simulink model "TestModel_V2_2024a"  (R2024a)
settings: Solver=FixedStepAuto  StartTime=0.0  StopTime=40  FixedStep=1e-6  RelTol=1e-3
values from neighbouring files (symbols this model uses):
  pmsm = mcb.getPMSMParameters('Teknic2310P')    [mcb_pmsm_foc_sensorless_f28379d_datascript.m]
  Ts = T_pwm    (= 5e-05)    [mcb_pmsm_foc_sensorless_f28379d_datascript.m]
  Ts_motor = T_pwm/2    (= 2.5e-05)    [mcb_pmsm_foc_sensorless_f28379d_datascript.m]
undefined symbols (not defined in the file or in its folder): DiscIntNeverNeededParam, IM, par_Ctrl_SpdRt
libraries: mcbcontrolslib x7, spsOnDelayLib x6, autolibim x3, spsCurrentMeasurementLib x2, spsDCVoltageSourceLib x2, spsVoltageMeasurementLib x2, spsTwoLevelConverterLib x2, spsThreePhaseVIMeasurementLib x2, spsTriangleGeneratorLib x2, spsUniversalBridgeLib x1, autolibpmsminterior x1, eePwmGeneratorTwoLevel x1
settings Model: SimulationMode=accelerator  PacingRate=1000  Creator=ckb527612  LastModifiedBy=ckb527612
settings ConfigComp: CovBoundaryAbsTol=1.0e-5
settings SimscapeCC: EditingMode=Restricted

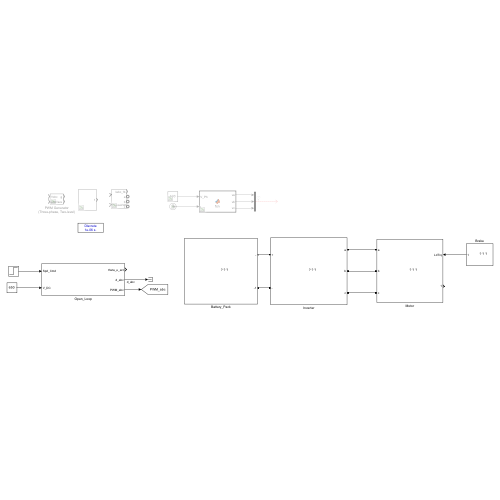
[thumbnail: Simulink's stored preview of the top-level diagram]
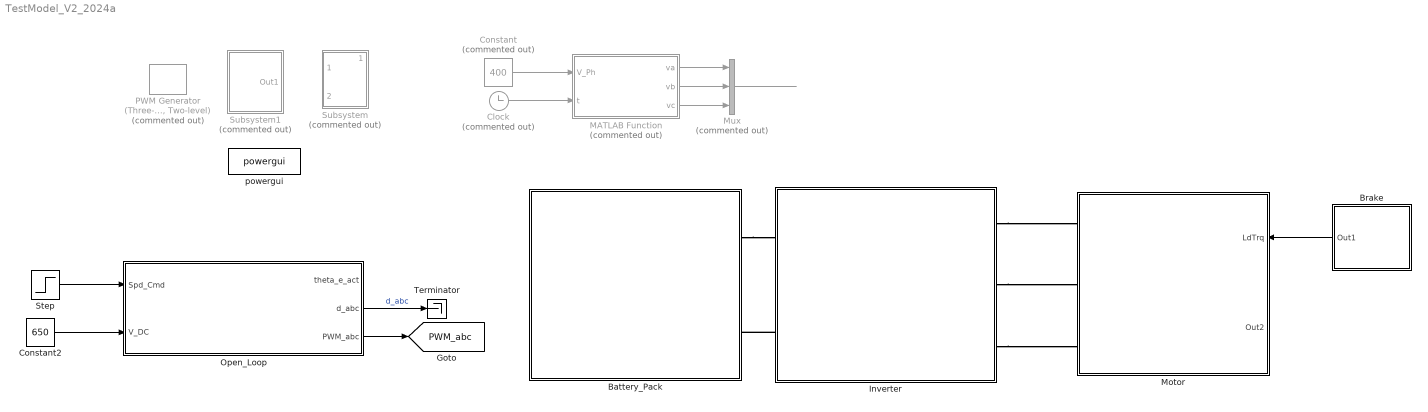
== system TestModel_V2_2024a ==
  Battery_Pack : Subsystem
      mask Display: image('battery_pack.jpg');
  Brake : Subsystem
      mask Display: image('brake-system-types-and-hydraulic-brake-parts-and-functions-6.png');
  Clock : Clock  Commented=on
  Constant : Constant  Commented=on  Value=400
  Constant2 : Constant  Value=650
  Inverter : Subsystem
      mask Display: image('inverter.jpg');
  MATLAB Function : MATLAB Function  Commented=on  TreatAsAtomicUnit=on
  Motor : Subsystem
      settings: PortSchema="{\"entries\":[{\"content\":{\"sides\":[{\"content\":{\"connectorIds\":[\"LConn1\",\"LConn2\",\"LConn3\"]},\"type\":\"ConnectorPlacement.EquallySpacedRectSide\",\"uuid\":\"ba224176-031b-46fb-9c66-bda2665a14bd\"},{\"content\":{\"connectorIds\":[\"In1\",\"Out1\"],\"side\":\"RIGHT\"},\"type\":\"ConnectorPlacement.EquallySpacedRectSide\",\"uuid\":\"afd0beac-69db-400a-8bb3-39f53f6dd0dc\"},{\"content\":{\"side\":\"TOP\"},\"type\":\"ConnectorPlacement.EquallySpacedRectSide\",\"uuid\":\"9d949d83-5907-4238-9cb9-0d10379fcdec\"}]},\"type\":\"ConnectorPlacement.EquallySpacedConnector\",\"uuid\":\"43d01ac6-0c0f-4af8-b336-a00f131902fe\"}],\"packageUris\":[\"http://schema.mathworks.com/mf0/Connector/R2020b\"],\"version\":\"1.0\"}"
      mask Display: image('Motor3.jpg');
  Mux : Mux  Commented=on  Inputs=3
  Open_Loop : Subsystem
  "PWM Generator (Three-phase, Two-level)" : eePwmGeneratorTwoLevel/PWM Generator (Three-phase, Two-level)  Commented=on  PWMMode=Continuous PWM (CPWM)  CPWMMode=SVM: space vector modulation  DPWMMode=60 DPWM: 60 degree discontinuous PWM  fsw=10e3  Ts=1e-6
      settings: LibrarySourceBlock=|
      | ee_sl_lib/Pulse Width
      | Modulation/PWM Generator
      | (Three-phase, Two-level)
  Step : Step  After=500
  Subsystem : Subsystem  Commented=on
  Subsystem1 : Subsystem  Commented=on
  Terminator : Terminator
  powergui : spspowerguiLib/powergui  Priority=1  SimulationMode=Discrete  SampleTime=1e-6  frequency=60  Iterations=50  frequencyindice=0  Pbase=100e6  ErrMax=1e-4  UnitsV=kV  UnitsW=MW  buscounter=0  FunctionMessages=off  echomessages=off  EnableUseOfTLC=off  CurrentSourceSwitches=off  DisableSnubberDevices=off  DisableRonSwitches=off  DisableVfSwitches=off  DisplayEquations=off  AutomaticDiscreteSolvers=off  SolverType=Tustin/Backward Euler (TBE)  Interpol=off  ExternalGateDelay=off  methode=off  Ts=100  x0status=blocks  SPID=on  SwTol=0  HookPort=off  NonlinearTolerance=1e-4  nMaxIteration=100  ContinueOnMaxIteration=off  RestoreLinks=warning  ResistiveCurrentMeasurement=off  Frange=[0:2:500]  Ylog=off  Xlog=on  ShowGrid=off  save=off  variable=ZData  structure=0  ZoomFFT=off  StartTime=0.0  cycles=1  DisplayStyle=1  fundamental=60  FreqAxis=off  MaxFrequency=1000  frequencyindicesteady=1  RmsSteady=1  display=off
  tag scope: PWM_abc=global
  wires:
  Constant/1 -> MATLAB Function/1(V_Ph)
  MATLAB Function/1(va) -> Mux/1
  MATLAB Function/2(vb) -> Mux/2
  MATLAB Function/3(vc) -> Mux/3
  Mux/1 -> ?
  Clock/1 -> MATLAB Function/2(t)
  Brake/1(Out1) -> Motor/1(LdTrq)
  Step/1 -> Open_Loop/1(Spd_Cmd)
  Constant2/1 -> Open_Loop/2(V_DC)
  Open_Loop/3(PWM_abc) -> [PWM_abc]
  Open_Loop/2(d_abc) -> Terminator/1  "d_abc"
  connections:
  Inverter/LConn2 -- Battery_Pack/RConn2
  Inverter/RConn2 -- Motor/LConn2
  Inverter/RConn1 -- Motor/LConn1
  Battery_Pack/RConn1 -- Inverter/LConn1
  Inverter/RConn3 -- Motor/LConn3

== system TestModel_V2_2024a/Battery_Pack ==
  Current Measurement : spsCurrentMeasurementLib/Current Measurement  PhasorSimulation=off  OutputType=Complex  PSBequivalent=0
  "V_in " : spsDCVoltageSourceLib/DC Voltage Source  Amplitude=650  Measurements=None
  Voltage Measurement : spsVoltageMeasurementLib/Voltage Measurement  PhasorSimulation=off  OutputType=Complex  PSBequivalent=0
  - : PMIOPort  Side=Right
  -1 : PMIOPort  Port=2  Side=Right
  tag scope: I_in=global, V_in=global
  wires:
  Current Measurement/1 -> [I_in]
  Voltage Measurement/1 -> [V_in]
  connections:
  Current Measurement/RConn1 -- -/RConn1
  Voltage Measurement/LConn1 -- Current Measurement/LConn1 -- "V_in "/RConn1
  "V_in "/LConn1 -- -1/RConn1 -- Voltage Measurement/LConn2

== system TestModel_V2_2024a/Brake ==
  Constant : Constant  Commented=on  Value=pmsm.LdTrq
  Data Type Conversion : DataTypeConversion  Commented=on  OutDataTypeStr=single  SaturateOnIntegerOverflow=off  RndMeth=Floor
  IIR Filter : mcbcontrolslib/IIR Filter  VariantControl=Low Pass Filter  VariantSelect=Low-pass  FilterConstantInputType=Specify via dialog  Filter_constant=0.001  InitialOutput=Specify via dialog  InitialOutputValue=0  ExternalReset=none  advancedSettings=off  Ts=50e-6  cutOff_freq=3.1863
  T_load : Step  Before=IM.Tshaft*0  After=IM.Tshaft*0.15  SampleTime=1e-6
  T_load1 : Step  Commented=on  Time=2.5  Before=pmsm.T_rated*0.1  After=pmsm.T_rated*0.5  SampleTime=Ts_motor
  Terminator : Terminator
  Out1 : Outport
  wires:
  Constant/1 -> Terminator/1
  T_load/1 -> IIR Filter/1
  IIR Filter/1 -> Out1/1

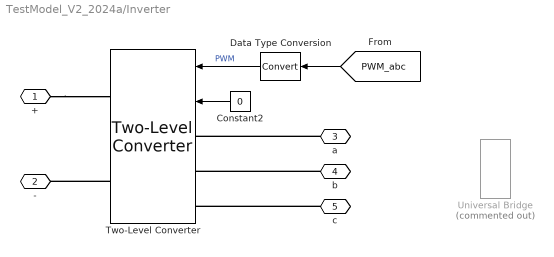
== system TestModel_V2_2024a/Inverter ==
  Constant2 : Constant  Value=0
  Data Type Conversion : DataTypeConversion  SaturateOnIntegerOverflow=off  RndMeth=Floor
  Two-Level Converter : spsTwoLevelConverterLib/Two-Level Converter  ModelType=Switching function  Ron=1e-3  Rs=1e6  Cs=inf  Vforward=[0,0]  Ron_Diode=1e-3  Rs_Diode=1e6  Cs_Diode=inf  Vf_Diode=0  Rs_CurrentSource=inf  Ron_ACsource=1e-3
  Universal Bridge : spsUniversalBridgeLib/Universal Bridge  Commented=on  Arms=3  SnubberResistance=1e5  SnubberCapacitance=inf  Device=IGBT / Diodes  Ron=1e-3  Lon=0  ForwardVoltages="[  0  0  ]"  ForwardVoltage=0  GTOparameters=[ 10e-6 , 20e-6 ]  IGBTparameters=[ 1e-6 , 2e-6 ]  Measurements=None  Measurements_2=None  converterType=Rectifier
  + : PMIOPort  Side=Left
  - : PMIOPort  Port=2  Side=Left
  a : PMIOPort  Port=3  Side=Right
  b : PMIOPort  Port=4  Side=Right
  c : PMIOPort  Port=5  Side=Right
  wires:
  Data Type Conversion/1 -> Two-Level Converter/1  "PWM"
  [PWM_abc] -> Data Type Conversion/1
  Constant2/1 -> Two-Level Converter/2
  connections:
  b/RConn1 -- Two-Level Converter/LConn2
  c/RConn1 -- Two-Level Converter/LConn3
  a/RConn1 -- Two-Level Converter/LConn1
  Two-Level Converter/RConn2 -- -/RConn1
  +/RConn1 -- Two-Level Converter/RConn1

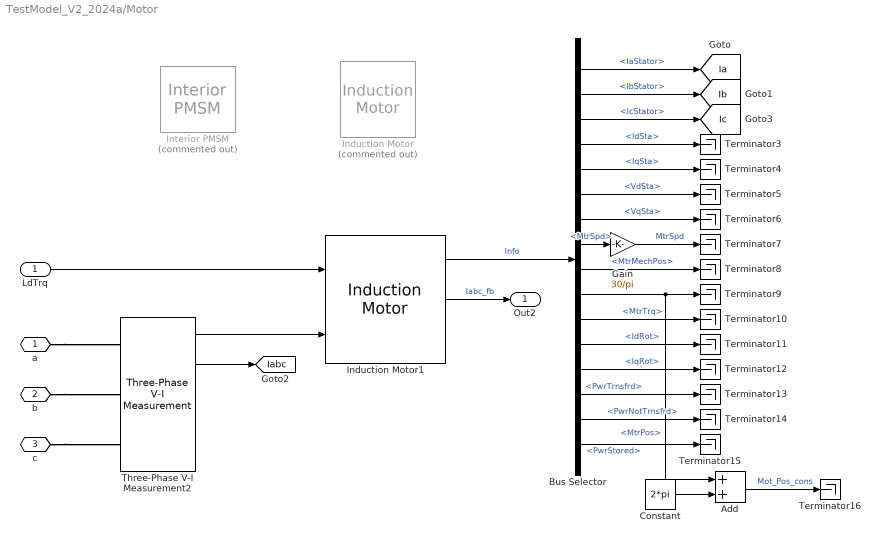
== system TestModel_V2_2024a/Motor ==
  LdTrq : Inport
  Add : Sum
  Bus Selector : BusSelector  OutputSignals=IaStator,IbStator,IcStator,IdSta,IqSta,VdSta,VqSta,MtrSpd,MtrMechPos,MtrPos,MtrTrq,IdRot,IqRot,PwrInfo.PwrTrnsfrd,PwrInfo.PwrNotTrnsfrd,PwrInfo.PwrStored
  Constant : Constant  Value=2*pi
  Gain : Gain  Gain=30/pi
  Induction Motor : autolibim/Induction Motor  Commented=on  sim_type=Discrete  Ts=0.001  port_config=Torque  P=2  Zs=[0.85 0.0139]  Zr="[0.55  0.0121]"  Lm=0.048  mechanical=[0.055 0.0078 0.5]  theta_init=0  omega_init=0  RefBlkName='autolibim/Induction Motor'  aMode=5
      settings: LibrarySourceBlock=mcblib/Electrical Systems/Motors/Induction Motor
  Induction Motor1 : autolibim/Induction Motor  sim_type=Discrete  Ts=1e-6  port_config=Torque  P=2  Zs=[3.14 0.0369]  Zr="[2.59  0.0369]"  Lm=0.527  mechanical=[0.01 0.00316 0.1]  theta_init=0  omega_init=0  RefBlkName='autolibim/Induction Motor'  aMode=5
      settings: LibrarySourceBlock=mcblib/Electrical Systems/Motors/Induction Motor
  Interior PMSM : autolibpmsminterior/Interior PMSM  Commented=on  port_config=Torque  sim_type=Continuous  Ts=0.001  FilePath=interiorpmsm_motordata.m  P=4  Rs=1.2  Ldq=[14.29e-3 23.15e-3]  KConstText=Permanent flux linkage constant (lambda_pm):  lambda_pm=0.5  Ke=159.9771  mechanical=[0.0045, 4.924e-4, 0]  idq0=[0 0]  theta_init=0  omega_init=0  KConst=0.1194  lambda_pm_calc=0.1194  Kt=1.323  RefBlkName='autolibpmsminterior/Interior PMSM'  aMode=1
      settings: LibrarySourceBlock=autolibemachines/Interior PMSM
  Terminator{3..16} (14 alike) : Terminator
  Three-Phase V-I Measurement2 : spsThreePhaseVIMeasurementLib/Three-Phase V-I Measurement  VoltageMeasurement=phase-to-phase  SetLabelV=off  LabelV=Vabc  Vpu=off  VpuLL=off  CurrentMeasurement=yes  SetLabelI=off  LabelI=Iabc  Ipu=off  Pbase=100e6  Vbase=500e3  OutputType=Complex  PhasorSimulation=off  PSBequivalent=0
  a : PMIOPort  Side=Left
  b : PMIOPort  Port=2  Side=Left
  c : PMIOPort  Port=3  Side=Left
  Out2 : Outport
  tag scope: Ia=global, Iabc=global, Ib=global, Ic=global
  wires:
  Three-Phase V-I Measurement2/2 -> [Iabc]
  LdTrq/1 -> Induction Motor1/1
  Three-Phase V-I Measurement2/1 -> Induction Motor1/2
  Induction Motor1/1 -> Bus Selector/1  "Info"
  Bus Selector/1 -> [Ia]  "<IaStator>"
  Bus Selector/5 -> Terminator4/1  "<IqSta>"
  Bus Selector/14 -> Terminator13/1  "<PwrTrnsfrd>"
  Bus Selector/6 -> Terminator5/1  "<VdSta>"
  Induction Motor1/2 -> Out2/1  "Iabc_fb"
  Gain/1 -> Terminator7/1  "MtrSpd"
  Bus Selector/12 -> Terminator11/1  "<IdRot>"
  Bus Selector/10 -> Add/1, Terminator9/1  "<MtrPos>"
  Bus Selector/11 -> Terminator10/1  "<MtrTrq>"
  Bus Selector/9 -> Terminator8/1  "<MtrMechPos>"
  Bus Selector/2 -> [Ib]  "<IbStator>"
  Bus Selector/4 -> Terminator3/1  "<IdSta>"
  Bus Selector/13 -> Terminator12/1  "<IqRot>"
  Bus Selector/15 -> Terminator14/1  "<PwrNotTrnsfrd>"
  Bus Selector/3 -> [Ic]  "<IcStator>"
  Bus Selector/16 -> Terminator15/1  "<PwrStored>"
  Bus Selector/7 -> Terminator6/1  "<VqSta>"
  Constant/1 -> Add/2
  Add/1 -> Terminator16/1  "Mot_Pos_cons"
  Bus Selector/8 -> Gain/1  "<MtrSpd>"
  connections:
  b/RConn1 -- Three-Phase V-I Measurement2/LConn2
  a/RConn1 -- Three-Phase V-I Measurement2/LConn1
  c/RConn1 -- Three-Phase V-I Measurement2/LConn3

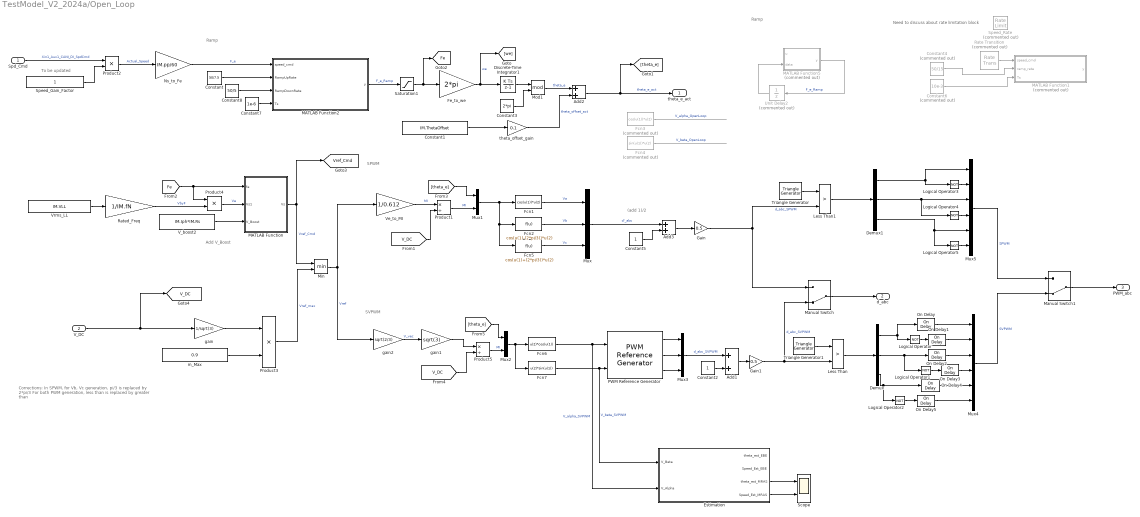
== system TestModel_V2_2024a/Open_Loop ==
  note: Corrections:
      | In SPWM, for Vb, Vc generation, pi/3 is replaced by 2*pi/3
      | For both PWM generation, less than is replaced by greater than
  note: Ramp
  note: SVPWM
  note: SPWM
  note: Add V_Boost
  note: Need to discuss about rate limitation block
  note: To be updated
  note: (add 1)/2
  note: Ramp
  Spd_Cmd : Inport
  V_DC : Inport  Port=2
  Add1 : Sum
  Add2 : Sum
  Add3 : Sum
  Constant : Constant  Value=50/7.5
  Constant1 : Constant  Value=IM.ThetaOffset
  Constant2 : Constant
  Constant3 : Constant  Value=2*pi  OutDataTypeStr=double
  Constant4 : Constant  Commented=on  Value=50/15
  Constant5 : Constant
  Constant6 : Constant  Commented=on  Value=10e-3
  Constant7 : Constant  Value=1e-6
  Constant8 : Constant  Value=50/5
  Demux : Demux  Outputs=3
  Demux1 : Demux  Outputs=3
  Discrete-Time Integrator1 : DiscreteIntegrator  SampleTime=-1  OutDataTypeStr=double  ICPrevOutput=DiscIntNeverNeededParam  ICPrevScaledInput=DiscIntNeverNeededParam
  Estimation : Subsystem
  Fcn1 : Fcn  Expr=cos(u(1))*u(2)
  Fcn2 : Fcn  Expr=cos(u(1)-(2*pi/3))*u(2)
  Fcn3 : Fcn  Commented=on  Expr=cos(u(1))*u(2)
  Fcn4 : Fcn  Commented=on  Expr=sin(u(1))*u(2)
  Fcn5 : Fcn  Expr=cos(u(1)+(2*pi/3))*u(2)
  Fcn6 : Fcn  Expr=u(2)*cos(u(1))
  Fcn7 : Fcn  Expr=u(2)*sin(u(1))
  Fe_to_we : Gain  Gain=2*pi
  Gain : Gain  Gain=0.5
  Gain1 : Gain  Gain=0.5
  Less Than : RelationalOperator  Operator=>  OutDataTypeStr=boolean  RndMeth=Simplest  InputSameDT=off
  Less Than1 : RelationalOperator  Operator=>  OutDataTypeStr=boolean  RndMeth=Simplest  InputSameDT=off
  Logical Operator{,1..5} (6 alike) : Logic  Operator=NOT  AllPortsSameDT=off  OutDataTypeStr=boolean
  MATLAB Function : MATLAB Function  TreatAsAtomicUnit=on
  MATLAB Function1 : MATLAB Function  Commented=on  TreatAsAtomicUnit=on
  MATLAB Function2 : MATLAB Function  TreatAsAtomicUnit=on
  MATLAB Function5 : MATLAB Function  Commented=on  TreatAsAtomicUnit=on
  Manual Switch : ManualSwitch  CurrentSetting=0
  Manual Switch1 : ManualSwitch  CurrentSetting=0
  Min : MinMax  Inputs=2
  Mod1 : Math  Operator=mod
  Mux : Mux  Inputs=3
  Mux1 : Mux  Inputs=2
  Mux2 : Mux  Inputs=2
  Mux3 : Mux  Inputs=3
  Mux4 : Mux  Inputs=6
  Mux5 : Mux  Inputs=6
  Ns_to_Fe : Gain  Gain=IM.pp/60
  On Delay{,1..5} (6 alike) : spsOnDelayLib/On Delay  DelayType=On delay  delay=3e-6  ic=0  Ts=1e-6
  PWM Reference Generator : mcbcontrolslib/PWM Reference Generator  inSignal=Valphabeta  modType=SVM: space vector modulation
      settings: LibrarySourceBlock=mcbhdllib/Controls/Math Transforms/PWM Reference Generator
  Product1 : Product  Inputs=*/
  Product2 : Product
  Product3 : Product
  Product4 : Product
  Product5 : Product  Inputs=*/
  Rate Transition : RateTransition  Commented=on  OutPortSampleTime=10e-3
  Rated_Freq : Gain  Gain=1/IM.fN  ParamDataTypeStr=double  OutDataTypeStr=double
  Saturation1 : Saturate  UpperLimit=50  LowerLimit=0
  Scope : Scope  NumInputPorts=2
  Speed_Gain_Factor : Constant
  Speed_Rate : RateLimiter  Commented=on  RisingSlewLimit=par_Ctrl_SpdRt  FallingSlewLimit=-par_Ctrl_SpdRt  SampleTimeMode=inherited
  Triangle Generator : spsTriangleGeneratorLib/Triangle Generator  Freq=10e3  Phase=0  Ts=1e-6
  Triangle Generator1 : spsTriangleGeneratorLib/Triangle Generator  Freq=10e3  Phase=0  Ts=1e-6
  Unit Delay2 : UnitDelay  Commented=on  SampleTime=-1  HasFrameUpgradeWarning=on
  V_boost2 : Constant  Value=IM.Iph*IM.Rs
  Ve_to_MI : Gain  Gain=1/0.612  ParamDataTypeStr=double  OutDataTypeStr=double
  Vrms_LL : Constant  Value=IM.VLL  OutDataTypeStr=double
  gain : Gain  Gain=1/sqrt(3)
  gain1 : Gain  Gain=sqrt(3)
  gain2 : Gain  Gain=sqrt(2/3)
  m_Max : Constant  Value=0.9
  theta_offset_gain : Gain  Gain=0.1
  theta_e_act : Outport
  d_abc : Outport  Port=2
  PWM_abc : Outport  Port=3
  tag scope: Fe=global, V_DC=global, Vref_Cmd=global
  wires:
  Product2/1 -> Ns_to_Fe/1  "Actual_Speed"
  Fe_to_we/1 -> Discrete-Time Integrator1/1, [we]  "we"
  Add2/1 -> theta_e_act/1, [theta_e]  "theta_e_act"
  Discrete-Time Integrator1/1 -> Mod1/1
  Mod1/1 -> Add2/1  "theta_e"
  Speed_Gain_Factor/1 -> Product2/2
  Ns_to_Fe/1 -> MATLAB Function2/1(speed_cmd)  "F_e"
  Constant3/1 -> Mod1/2
  theta_offset_gain/1 -> Add2/2  "theta_offset_act"
  Spd_Cmd/1 -> Product2/1  "Xin1_Aux1_CANI_DI_SpdCmd"
  Constant1/1 -> theta_offset_gain/1
  Vrms_LL/1 -> Rated_Freq/1
  Rated_Freq/1 -> Product4/2  "VbyF"
  [Fe] -> Product4/1, MATLAB Function/1(fe)
  Product4/1 -> MATLAB Function/2(Vs1)  "Ve"
  Product1/1 -> Mux1/2  "MI"
  [theta_e] -> Mux1/1
  Fcn3/1 -> ?  "V_alpha_OpenLoop"
  Fcn4/1 -> ?  "V_beta_OpenLoop"
  V_boost2/1 -> MATLAB Function/3(V_Boost)
  MATLAB Function/1(Vs) -> Min/1, [Vref_Cmd]  "Vref_Cmd"
  V_DC/1 -> [V_DC], gain/1
  Ve_to_MI/1 -> Product1/1  "MI"
  Mux1/1 -> Fcn5/1, Fcn2/1, Fcn1/1
  Fcn1/1 -> Mux/1  "Va"
  Fcn2/1 -> Mux/2  "Vb"
  Fcn5/1 -> Mux/3  "Vc"
  Constant5/1 -> Add3/2
  Add3/1 -> Gain/1
  Mux/1 -> Add3/1  "d'_abc"
  Manual Switch/1 -> d_abc/1
  m_Max/1 -> Product3/2
  gain/1 -> Product3/1
  Product3/1 -> Min/2  "Vref_max"
  Min/1 -> gain2/1, Ve_to_MI/1  "Vref"
  [V_DC] -> Product1/2
  gain1/1 -> Product5/1
  [V_DC] -> Product5/2
  Product5/1 -> Mux2/2  "MI"
  [theta_e] -> Mux2/1
  Mux2/1 -> Fcn6/1, Fcn7/1
  Fcn6/1 -> Estimation/2(V_Alpha), PWM Reference Generator/1  "V_alpha_SVPWM"
  Fcn7/1 -> Estimation/1(V_Beta), PWM Reference Generator/2  "V_beta_SVPWM"
  PWM Reference Generator/1 -> Mux3/1
  PWM Reference Generator/2 -> Mux3/2
  PWM Reference Generator/3 -> Mux3/3
  Gain1/1 -> Less Than/2, Manual Switch/2  "d_abc_SVPWM"
  Gain/1 -> Less Than1/2, Manual Switch/1  "d_abc_SPWM"
  gain2/1 -> gain1/1  "V_vec"
  Add1/1 -> Gain1/1
  Constant2/1 -> Add1/2
  Mux3/1 -> Add1/1  "d_abc_SVPWM"
  Demux/1 -> Logical Operator/1, On Delay/1
  Logical Operator/1 -> On Delay1/1
  Logical Operator1/1 -> On Delay3/1
  Demux/2 -> On Delay2/1, Logical Operator1/1
  On Delay5/1 -> Mux4/6
  Demux/3 -> On Delay4/1, Logical Operator2/1
  Mux4/1 -> Manual Switch1/2  "SVPWM"
  Mux5/1 -> Manual Switch1/1  "SPWM"
  Demux1/3 -> Mux5/5, Logical Operator5/1
  Demux1/2 -> Mux5/3, Logical Operator4/1
  Demux1/1 -> Mux5/1, Logical Operator3/1
  Logical Operator3/1 -> Mux5/2
  Logical Operator4/1 -> Mux5/4
  Logical Operator5/1 -> Mux5/6
  Manual Switch1/1 -> PWM_abc/1
  Triangle Generator1/1 -> Less Than/1
  Less Than/1 -> Demux/1
  Triangle Generator/1 -> Less Than1/1
  Less Than1/1 -> Demux1/1
  On Delay/1 -> Mux4/1
  On Delay1/1 -> Mux4/2
  On Delay2/1 -> Mux4/3
  On Delay4/1 -> Mux4/5
  On Delay3/1 -> Mux4/4
  Logical Operator2/1 -> On Delay5/1
  Saturation1/1 -> Fe_to_we/1, [Fe]
  Constant6/1 -> MATLAB Function1/3(Ts)
  Rate Transition/1 -> MATLAB Function1/1(speed_cmd)
  Constant4/1 -> MATLAB Function1/2(ramp_rate)
  ? -> Rate Transition/1
  Constant/1 -> MATLAB Function2/2(RampUpRate)
  Constant8/1 -> MATLAB Function2/3(RampDownRate)
  Constant7/1 -> MATLAB Function2/4(Ts)
  MATLAB Function5/1(y) -> Unit Delay2/1  "F_e_Ramp"
  Unit Delay2/1 -> MATLAB Function5/2(data)
  MATLAB Function2/1(y) -> Saturation1/1  "F_e_Ramp"
  Estimation/3(theta_est_MRAS) -> Scope/1
  Estimation/4(Speed_Est_MRAS) -> Scope/2

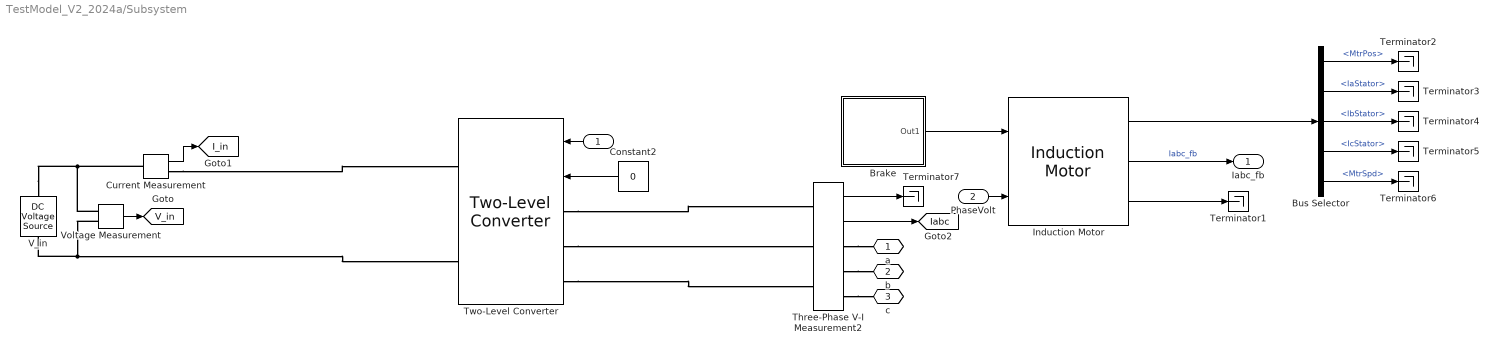
== system TestModel_V2_2024a/Subsystem ==
  "  " : Inport
  PhaseVolt : Inport  Port=2
  Brake : Subsystem
      mask Display: image('brake-system-types-and-hydraulic-brake-parts-and-functions-6.png');
  Bus Selector : BusSelector  OutputSignals=MtrPos,IaStator,IbStator,IcStator,MtrSpd
  Constant2 : Constant  Value=0
  Current Measurement : spsCurrentMeasurementLib/Current Measurement  PhasorSimulation=off  OutputType=Complex  PSBequivalent=0
  Induction Motor : autolibim/Induction Motor  sim_type=Discrete  Ts=0.001  port_config=Torque  P=2  Zs=[0.85 0.0139]  Zr="[0.55  0.0121]"  Lm=0.048  mechanical=[0.055 0.0078 0.5]  theta_init=0  omega_init=0  RefBlkName='autolibim/Induction Motor'  aMode=5
      settings: LibrarySourceBlock=mcblib/Electrical Systems/Motors/Induction Motor
  Terminator{1..7} (7 alike) : Terminator
  Three-Phase V-I Measurement2 : spsThreePhaseVIMeasurementLib/Three-Phase V-I Measurement  VoltageMeasurement=phase-to-phase  SetLabelV=off  LabelV=Vabc  Vpu=off  VpuLL=off  CurrentMeasurement=yes  SetLabelI=off  LabelI=Iabc  Ipu=off  Pbase=100e6  Vbase=500e3  OutputType=Complex  PhasorSimulation=off  PSBequivalent=0
  Two-Level Converter : spsTwoLevelConverterLib/Two-Level Converter  ModelType=Switching devices  Ron=1e-3  Rs=1e6  Cs=inf  Vforward=[0,0]  Ron_Diode=1e-3  Rs_Diode=1e6  Cs_Diode=inf  Vf_Diode=1e-3  Rs_CurrentSource=inf  Ron_ACsource=1e-3
      settings: LibrarySourceBlock=sps_lib/Power Electronics/Two-Level Converter
  "V_in " : spsDCVoltageSourceLib/DC Voltage Source  Amplitude=650  Measurements=None
  Voltage Measurement : spsVoltageMeasurementLib/Voltage Measurement  PhasorSimulation=off  OutputType=Complex  PSBequivalent=0
  a : PMIOPort  Side=Right
  b : PMIOPort  Port=2  Side=Right
  c : PMIOPort  Port=3  Side=Right
  Iabc_fb : Outport
  tag scope: I_in=global, Iabc=global, V_in=global
  wires:
  Bus Selector/2 -> Terminator3/1  "<IaStator>"
  Voltage Measurement/1 -> [V_in]
  Bus Selector/1 -> Terminator2/1  "<MtrPos>"
  Three-Phase V-I Measurement2/2 -> [Iabc]
  Brake/1(Out1) -> Induction Motor/1
  Induction Motor/2 -> Iabc_fb/1  "Iabc_fb"
  Bus Selector/5 -> Terminator6/1  "<MtrSpd>"
  Current Measurement/1 -> [I_in]
  Bus Selector/3 -> Terminator4/1  "<IbStator>"
  "  "/1 -> Two-Level Converter/1
  Induction Motor/1 -> Bus Selector/1
  Three-Phase V-I Measurement2/1 -> Terminator7/1
  Bus Selector/4 -> Terminator5/1  "<IcStator>"
  Constant2/1 -> Two-Level Converter/2
  Induction Motor/3 -> Terminator1/1
  PhaseVolt/1 -> Induction Motor/2
  connections:
  Two-Level Converter/LConn2 -- Three-Phase V-I Measurement2/LConn2
  Voltage Measurement/LConn2 -- "V_in "/LConn1 -- Two-Level Converter/RConn2
  Two-Level Converter/LConn1 -- Three-Phase V-I Measurement2/LConn1
  Three-Phase V-I Measurement2/RConn3 -- c/RConn1
  Two-Level Converter/LConn3 -- Three-Phase V-I Measurement2/LConn3
  "V_in "/RConn1 -- Voltage Measurement/LConn1 -- Current Measurement/LConn1
  Current Measurement/RConn1 -- Two-Level Converter/RConn1
  Three-Phase V-I Measurement2/RConn2 -- b/RConn1
  Three-Phase V-I Measurement2/RConn1 -- a/RConn1

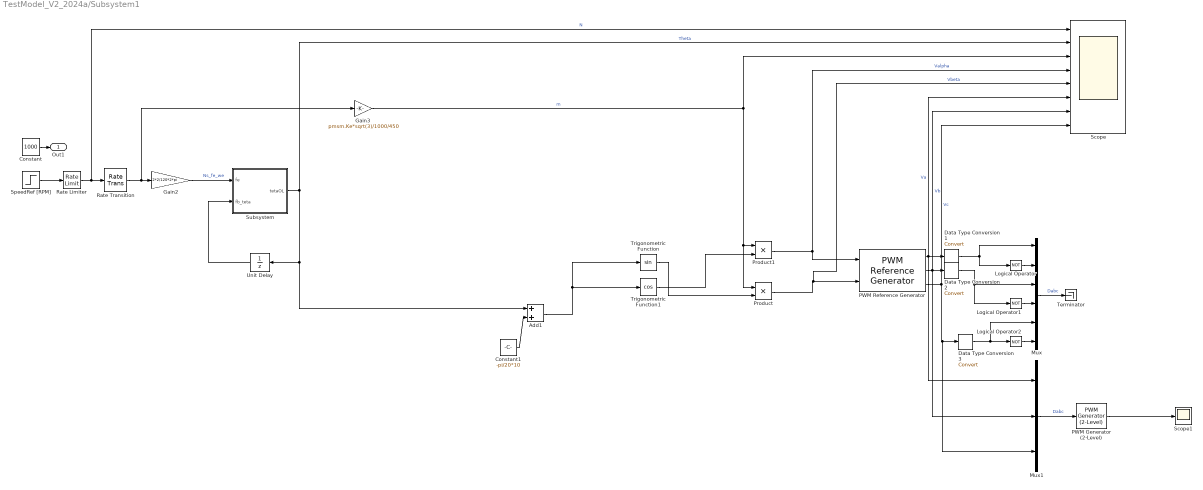
== system TestModel_V2_2024a/Subsystem1 ==
  Add1 : Sum
  Constant : Constant  Value=1000
  Constant1 : Constant  Value=-pi/20*10
  Data Type Conversion1 : DataTypeConversion  SaturateOnIntegerOverflow=off  RndMeth=Floor
  Data Type Conversion2 : DataTypeConversion  SaturateOnIntegerOverflow=off  RndMeth=Floor
  Data Type Conversion3 : DataTypeConversion  SaturateOnIntegerOverflow=off  RndMeth=Floor
  Gain2 : Gain  Gain=2*2/120*2*pi
  Gain3 : Gain  Gain=pmsm.Ke*sqrt(3)/1000/450
  Logical Operator : Logic  Operator=NOT  AllPortsSameDT=off  OutDataTypeStr=boolean
  Logical Operator1 : Logic  Operator=NOT  AllPortsSameDT=off  OutDataTypeStr=boolean
  Logical Operator2 : Logic  Operator=NOT  AllPortsSameDT=off  OutDataTypeStr=boolean
  Mux : Mux  Inputs=6
  Mux1 : Mux  Inputs=3
  PWM Generator (2-Level) : spsPWMGenerator2LevelLib/PWM Generator (2-Level)  ModulatorType=Three-phase bridge (6 pulses)  ModulatorMode=Unsynchronized  Fc=10000  Pc=90  nF=27  MinMax="[ -1  1 ]"  SamplingTechnique=Natural  ModulatingSignals=off  m=0.8  Freq=60  Phase=0  Ts=1e-6  ShowCarrierOutport=off
  PWM Reference Generator : mcbcontrolslib/PWM Reference Generator  inSignal=Valphabeta  modType=SVM: space vector modulation
      settings: LibrarySourceBlock=mcblib/Controls/Math Transforms/PWM Reference Generator
  Product : Product
  Product1 : Product
  Rate Limiter : RateLimiter  RisingSlewLimit=1000  SampleTimeMode=inherited
  Rate Transition : RateTransition  OutPortSampleTime=10e-5
  Scope : Scope  NumInputPorts=8
  Scope1 : Scope
  SpeedRef [RPM] : Step  Time=2  Before=500  After=1000  OutDataTypeStr=single  SampleTime=Ts
  Subsystem : Subsystem
  Terminator : Terminator
  Trigonometric Function : Trigonometry
  Trigonometric Function1 : Trigonometry  Operator=cos
  Unit Delay : UnitDelay  SampleTime=-1  HasFrameUpgradeWarning=on
  Out1 : Outport
  wires:
  SpeedRef [RPM]/1 -> Rate Limiter/1
  PWM Reference Generator/1 -> Mux1/1, Scope/6, Data Type Conversion1/1  "Va"
  PWM Reference Generator/2 -> Mux1/2, Scope/7, Data Type Conversion2/1  "Vb"
  Gain3/1 -> Product/1, Product1/1, Scope/3  "m"
  Gain2/1 -> Subsystem/1(fe)  "Ns_fe_we"
  Constant1/1 -> Add1/2
  Logical Operator2/1 -> Mux/6
  Data Type Conversion3/1 -> Mux/5, Logical Operator2/1
  Rate Transition/1 -> Gain3/1, Gain2/1
  Data Type Conversion2/1 -> Logical Operator1/1, Mux/3
  Product/1 -> Scope/5, PWM Reference Generator/2  "Vbeta"
  Trigonometric Function/1 -> Product/2
  Logical Operator/1 -> Mux/2
  Unit Delay/1 -> Subsystem/2(fb_teta)
  Mux/1 -> Terminator/1  "Dabc"
  Data Type Conversion1/1 -> Logical Operator/1, Mux/1
  Rate Limiter/1 -> Scope/1, Rate Transition/1  "N"
  Logical Operator1/1 -> Mux/4
  Add1/1 -> Trigonometric Function1/1, Trigonometric Function/1
  Product1/1 -> Scope/4, PWM Reference Generator/1  "Valpha"
  Trigonometric Function1/1 -> Product1/2
  PWM Reference Generator/3 -> Scope/8, Mux1/3, Data Type Conversion3/1  "Vc"
  PWM Generator (2-Level)/1 -> Scope1/1
  Constant/1 -> Out1/1
  Mux1/1 -> PWM Generator (2-Level)/1  "Dabc"
  Subsystem/1(tetaOL) -> Add1/1, Unit Delay/1, Scope/2  "Theta"

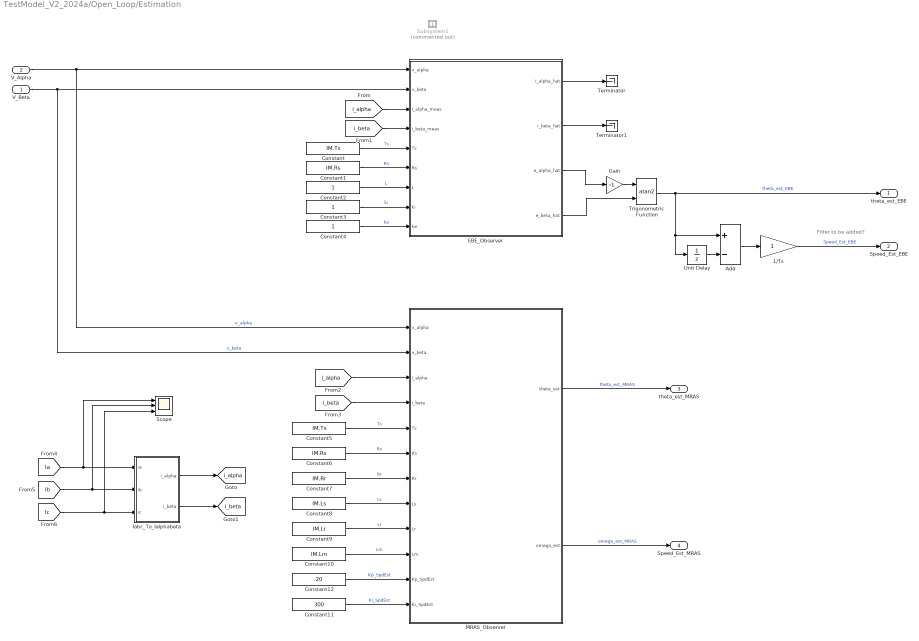
== system TestModel_V2_2024a/Open_Loop/Estimation ==
  note: Filter to be added?
  V_Beta : Inport
  V_Alpha : Inport  Port=2
  1/Ts : Gain
  Add : Sum  Inputs=+-
  Constant : Constant  Value=IM.Ts
  Constant1 : Constant  Value=IM.Rs
  Constant10 : Constant  Value=IM.Lm
  Constant11 : Constant  Value=300
  Constant12 : Constant  Value=20
  Constant2 : Constant
  Constant3 : Constant
  Constant4 : Constant
  Constant5 : Constant  Value=IM.Ts
  Constant6 : Constant  Value=IM.Rs
  Constant7 : Constant  Value=IM.Rr
  Constant8 : Constant  Value=IM.Ls
  Constant9 : Constant  Value=IM.Lr
  EBE_Observer : MATLAB Function  TreatAsAtomicUnit=on
  Gain : Gain  Gain=-1
  Iabc_To_Ialphabeta : Subsystem
  MRAS_Observer : MATLAB Function  TreatAsAtomicUnit=on
  Scope : Scope  NumInputPorts=3
  Subsystem1 : Subsystem  Commented=on
  Terminator : Terminator
  Terminator1 : Terminator
  Trigonometric Function : Trigonometry  Operator=atan2
  Unit Delay : UnitDelay  SampleTime=-1  HasFrameUpgradeWarning=on
  theta_est_EBE : Outport  VectorParamsAs1DForOutWhenUnconnected=off
  Speed_Est_EBE : Outport  Port=2  VectorParamsAs1DForOutWhenUnconnected=off
  theta_est_MRAS : Outport  Port=3  VectorParamsAs1DForOutWhenUnconnected=off
  Speed_Est_MRAS : Outport  Port=4  VectorParamsAs1DForOutWhenUnconnected=off
  tag scope: i_alpha=global, i_beta=global
  wires:
  [Ia] -> Scope/1, Iabc_To_Ialphabeta/1(ia)
  [Ib] -> Scope/2, Iabc_To_Ialphabeta/2(ib)
  [Ic] -> Scope/3, Iabc_To_Ialphabeta/3(ic)
  Iabc_To_Ialphabeta/1(i_alpha) -> [i_alpha]
  Iabc_To_Ialphabeta/2(i_beta) -> [i_beta]
  V_Alpha/1 -> MRAS_Observer/1(v_alpha), EBE_Observer/1(v_alpha)  "v_alpha"
  V_Beta/1 -> MRAS_Observer/2(v_beta), EBE_Observer/2(v_beta)  "v_beta"
  Constant/1 -> EBE_Observer/5(Ts)  "Ts"
  Constant1/1 -> EBE_Observer/6(Rs)  "Rs"
  Constant2/1 -> EBE_Observer/7(L)  "L"
  Constant3/1 -> EBE_Observer/8(ki)  "ki"
  Constant4/1 -> EBE_Observer/9(ke)  "ke"
  EBE_Observer/3(e_alpha_hat) -> Gain/1
  Gain/1 -> Trigonometric Function/1
  EBE_Observer/4(e_beta_hat) -> Trigonometric Function/2
  Trigonometric Function/1 -> Unit Delay/1, Add/1, theta_est_EBE/1  "theta_est_EBE"
  Unit Delay/1 -> Add/2
  Add/1 -> 1/Ts/1
  1/Ts/1 -> Speed_Est_EBE/1  "Speed_Est_EBE"
  EBE_Observer/1(i_alpha_hat) -> Terminator/1
  EBE_Observer/2(i_beta_hat) -> Terminator1/1
  [i_alpha] -> EBE_Observer/3(i_alpha_meas)
  [i_beta] -> EBE_Observer/4(i_beta_meas)
  [i_alpha] -> MRAS_Observer/3(i_alpha)
  [i_beta] -> MRAS_Observer/4(i_beta)
  Constant9/1 -> MRAS_Observer/9(Lr)  "Lr"
  Constant7/1 -> MRAS_Observer/7(Rr)  "Rr"
  Constant6/1 -> MRAS_Observer/6(Rs)  "Rs"
  Constant5/1 -> MRAS_Observer/5(Ts)  "Ts"
  Constant10/1 -> MRAS_Observer/10(Lm)  "Lm"
  Constant12/1 -> MRAS_Observer/11(Kp_SpdEst)  "Kp_SpdEst"
  Constant11/1 -> MRAS_Observer/12(Ki_SpdEst)  "Ki_SpdEst"
  MRAS_Observer/1(theta_est) -> theta_est_MRAS/1  "theta_est_MRAS"
  MRAS_Observer/2(omega_est) -> Speed_Est_MRAS/1  "omega_est_MRAS"
  Constant8/1 -> MRAS_Observer/8(Ls)  "Ls"

== system TestModel_V2_2024a/Subsystem/Brake ==
  Constant : Constant  Commented=on  Value=pmsm.LdTrq
  Data Type Conversion : DataTypeConversion  Commented=on  OutDataTypeStr=single  SaturateOnIntegerOverflow=off  RndMeth=Floor
  IIR Filter : mcbcontrolslib/IIR Filter  VariantControl=Low Pass Filter  VariantSelect=Low-pass  FilterConstantInputType=Specify via dialog  Filter_constant=0.001  InitialOutput=Specify via dialog  InitialOutputValue=0  ExternalReset=none  advancedSettings=off  Ts=50e-6  cutOff_freq=3.1863
  T_load : Step  Time=2.5  Before=pmsm.T_rated*0  After=pmsm.T_rated*0.1  SampleTime=Ts_motor
  T_load1 : Step  Commented=on  Time=2.5  Before=pmsm.T_rated*0.1  After=pmsm.T_rated*0.5  SampleTime=Ts_motor
  Terminator : Terminator
  Out1 : Outport
  wires:
  Constant/1 -> Terminator/1
  T_load/1 -> IIR Filter/1
  IIR Filter/1 -> Out1/1

== system TestModel_V2_2024a/Subsystem1/Subsystem ==
  fe : Inport
  fb_teta : Inport  Port=2
  2pi : Constant  Value=2*pi
  Discrete-Time Integrator : DiscreteIntegrator  ExternalReset=rising  SampleTime=-1  LimitOutput=on  UpperSaturationLimit=2*pi  LowerSaturationLimit=0  ICPrevOutput=DiscIntNeverNeededParam  ICPrevScaledInput=DiscIntNeverNeededParam
  Equal : RelationalOperator  OutDataTypeStr=boolean  RndMeth=Simplest  InputSameDT=off
  tetaOL : Outport
  wires:
  fb_teta/1 -> Equal/1
  Equal/1 -> Discrete-Time Integrator/2
  2pi/1 -> Equal/2
  Discrete-Time Integrator/1 -> tetaOL/1  "tetaOL"
  fe/1 -> Discrete-Time Integrator/1

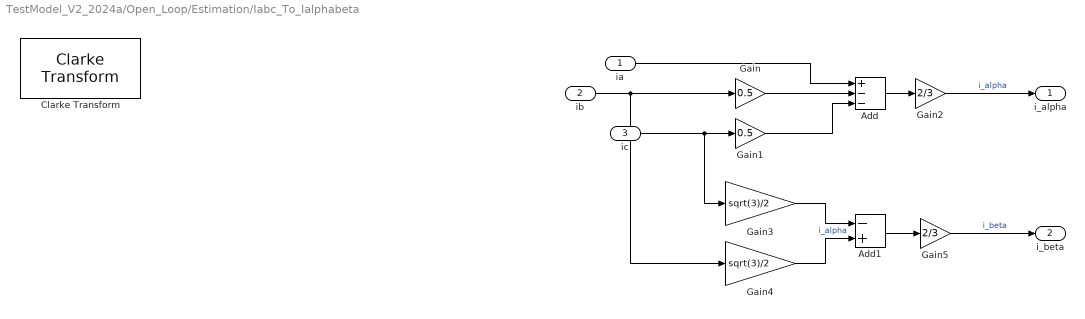
== system TestModel_V2_2024a/Open_Loop/Estimation/Iabc_To_Ialphabeta ==
  ia : Inport
  ib : Inport  Port=2
  ic : Inport  Port=3
  Add : Sum  Inputs=+--
  Add1 : Sum  Inputs=-+
  Clarke Transform : mcbcontrolslib/Clarke Transform  VariantControl=Variant2  EnPowerInv=off  PhaseInput=Two inputs
      settings: LibrarySourceBlock=mcbhdllib/Controls/Math Transforms/Clarke Transform
  Gain : Gain  Gain=0.5
  Gain1 : Gain  Gain=0.5
  Gain2 : Gain  Gain=2/3
  Gain3 : Gain  Gain=sqrt(3)/2
  Gain4 : Gain  Gain=sqrt(3)/2
  Gain5 : Gain  Gain=2/3
  i_alpha : Outport
  i_beta : Outport  Port=2
  wires:
  Gain3/1 -> Add1/1
  Gain/1 -> Add/2
  ib/1 -> Gain4/1, Gain/1
  Gain5/1 -> i_beta/1  "i_beta"
  ic/1 -> Gain3/1, Gain1/1
  Gain1/1 -> Add/3
  Add1/1 -> Gain5/1
  Add/1 -> Gain2/1
  Gain4/1 -> Add1/2  "i_alpha"
  ia/1 -> Add/1
  Gain2/1 -> i_alpha/1  "i_alpha"

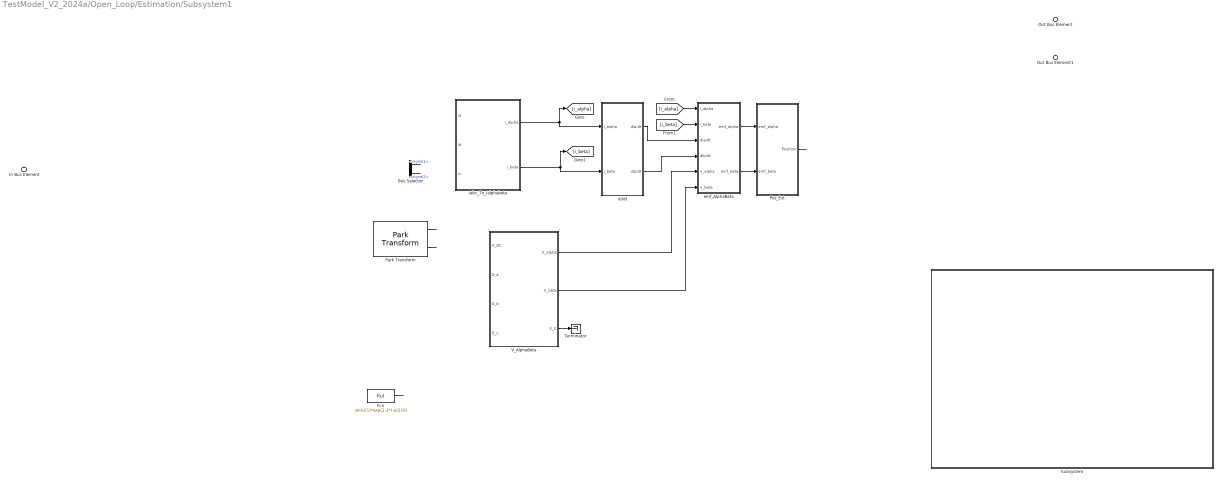
== system TestModel_V2_2024a/Open_Loop/Estimation/Subsystem1 ==
  In Bus Element : Inport  PortName=Ctrl_ScaledISR_In  Element=signal1
  Bus Selector : BusSelector  OutputSignals=signal1,signal2
  Fcn : Fcn  Expr=sin(u(1)*exp(2.3*(-u(2))))
  Iabc_To_Ialphabeta : Subsystem
  Park Transform : mcbcontrolslib/Park Transform  AxisAlignment=D-axis  PhaseInput=Two inputs  ThetaInput=Sine and Cosine electrical position  AngleInput=Per-unit  N_points=1024
      settings: LibrarySourceBlock=mcbhdllib/Controls/Math Transforms/Park Transform
  Pos_Est : Subsystem
  Subsystem : Subsystem
  Terminator : Terminator
  V_AlphaBeta : Subsystem
  di/dt : Subsystem
  emf_AlphaBeta : Subsystem
  Out Bus Element : Outport  PortName=Position_Est  Element=signal1
  Out Bus Element1 : Outport  Port=2  PortName=Speed_Est  Element=signal1
  wires:
  di/dt/1(dia/dt) -> emf_AlphaBeta/3(dia/dt)
  Iabc_To_Ialphabeta/1(i_alpha) -> di/dt/1(i_alpha), [i_alpha]
  emf_AlphaBeta/2(emf_beta) -> Pos_Est/2(emf_beta)
  di/dt/2(dib/dt) -> emf_AlphaBeta/4(dib/dt)
  emf_AlphaBeta/1(emf_alpha) -> Pos_Est/1(emf_alpha)
  V_AlphaBeta/3(V_C) -> Terminator/1
  [i_beta] -> emf_AlphaBeta/2(i_beta)
  [i_alpha] -> emf_AlphaBeta/1(i_alpha)
  V_AlphaBeta/2(V_beta) -> emf_AlphaBeta/6(v_beta)
  ? -> V_AlphaBeta/3(D_b)
  ? -> V_AlphaBeta/1(V_DC)
  V_AlphaBeta/1(V_alpha) -> emf_AlphaBeta/5(v_alpha)
  Iabc_To_Ialphabeta/2(i_beta) -> di/dt/2(i_beta), [i_beta]
  Park Transform/2 -> ?
  Fcn/1 -> ?
  ? -> Iabc_To_Ialphabeta/2(ib)
  Pos_Est/1(Position) -> ?
  ? -> Iabc_To_Ialphabeta/3(ic)
  ? -> Iabc_To_Ialphabeta/1(ia)
  ? -> V_AlphaBeta/4(D_c)
  ? -> V_AlphaBeta/2(D_a)
  Bus Selector/1 -> ?  "<signal1>"
  ? -> Fcn/1
  Park Transform/1 -> ?
  Bus Selector/2 -> ?  "<signal2>"

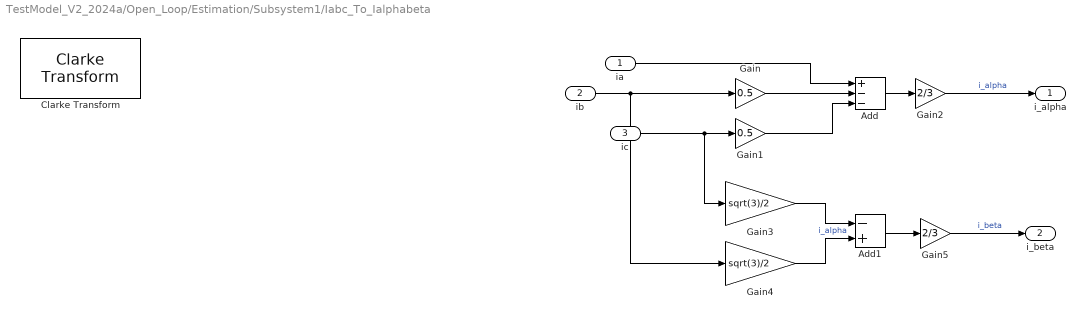
== system TestModel_V2_2024a/Open_Loop/Estimation/Subsystem1/Iabc_To_Ialphabeta ==
  ia : Inport
  ib : Inport  Port=2
  ic : Inport  Port=3
  Add : Sum  Inputs=+--
  Add1 : Sum  Inputs=-+
  Clarke Transform : mcbcontrolslib/Clarke Transform  VariantControl=Variant2  EnPowerInv=off  PhaseInput=Two inputs
      settings: LibrarySourceBlock=mcbhdllib/Controls/Math Transforms/Clarke Transform
  Gain : Gain  Gain=0.5
  Gain1 : Gain  Gain=0.5
  Gain2 : Gain  Gain=2/3
  Gain3 : Gain  Gain=sqrt(3)/2
  Gain4 : Gain  Gain=sqrt(3)/2
  Gain5 : Gain  Gain=2/3
  i_alpha : Outport
  i_beta : Outport  Port=2
  wires:
  Gain3/1 -> Add1/1
  Gain/1 -> Add/2
  ib/1 -> Gain4/1, Gain/1
  Gain5/1 -> i_beta/1  "i_beta"
  ic/1 -> Gain3/1, Gain1/1
  Gain1/1 -> Add/3
  Add1/1 -> Gain5/1
  Add/1 -> Gain2/1
  Gain4/1 -> Add1/2  "i_alpha"
  ia/1 -> Add/1
  Gain2/1 -> i_alpha/1  "i_alpha"

== system TestModel_V2_2024a/Open_Loop/Estimation/Subsystem1/Pos_Est ==
  emf_alpha : Inport
  emf_beta : Inport  Port=2
  Gain : Gain
  Trigonometric Function : Trigonometry  Operator=atan2
  Position : Outport
  wires:
  emf_alpha/1 -> Gain/1
  Gain/1 -> Trigonometric Function/1
  emf_beta/1 -> Trigonometric Function/2
  Trigonometric Function/1 -> Position/1

== system TestModel_V2_2024a/Open_Loop/Estimation/Subsystem1/Subsystem ==
  1/L : Gain
  Add : Sum  Inputs=+-
  Add1 : Sum
  Add2 : Sum  Inputs=+--
  Add3 : Sum  Inputs=+-
  Ke : Gain
  Ki : Gain
  Rs : Gain
  Unit Delay : UnitDelay  SampleTime=-1  HasFrameUpgradeWarning=on
  wires:
  ? -> Add/1  "i_alpha_meas"
  ? -> Unit Delay/1, Rs/1, Add/2  "i_alpha_est"
  Add/1 -> Ki/1, Ke/1  "i_alpha_tilde"
  Ke/1 -> ?  "d(e_alpha_est)/dt"
  Ki/1 -> Add1/1  "d(e_alpha_est)/dt"
  Add1/1 -> Add3/1  "d(i_alpha_est)/dt"
  ? -> Add2/1  "v_alpha"
  Rs/1 -> Add2/2
  ? -> Add2/3  "e_alpha_est"
  Add2/1 -> 1/L/1
  1/L/1 -> Add1/2
  Unit Delay/1 -> Add3/2

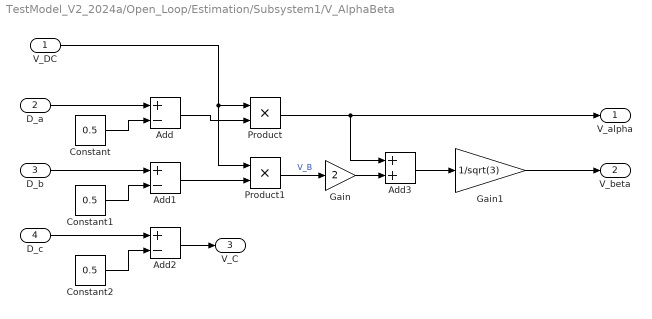
== system TestModel_V2_2024a/Open_Loop/Estimation/Subsystem1/V_AlphaBeta ==
  V_DC : Inport
  D_a : Inport  Port=2
  D_b : Inport  Port=3
  D_c : Inport  Port=4
  Add : Sum  Inputs=+-
  Add1 : Sum  Inputs=+-
  Add2 : Sum  Inputs=+-
  Add3 : Sum
  Constant : Constant  Value=0.5
  Constant1 : Constant  Value=0.5
  Constant2 : Constant  Value=0.5
  Gain : Gain  Gain=2
  Gain1 : Gain  Gain=1/sqrt(3)
  Product : Product
  Product1 : Product
  V_alpha : Outport
  V_beta : Outport  Port=2
  V_C : Outport  Port=3
  wires:
  D_a/1 -> Add/1
  Constant/1 -> Add/2
  D_b/1 -> Add1/1
  Constant1/1 -> Add1/2
  D_c/1 -> Add2/1
  Constant2/1 -> Add2/2
  Add/1 -> Product/2
  V_DC/1 -> Product1/1, Product/1
  Product/1 -> Add3/1, V_alpha/1
  Add1/1 -> Product1/2
  Add2/1 -> V_C/1
  Product1/1 -> Gain/1  "V_B"
  Gain/1 -> Add3/2
  Add3/1 -> Gain1/1
  Gain1/1 -> V_beta/1

== system TestModel_V2_2024a/Open_Loop/Estimation/Subsystem1/di//dt ==
  i_alpha : Inport
  i_beta : Inport  Port=2
  Subsystem : Subsystem
  Subsystem1 : Subsystem
  dia/dt : Outport
  dib/dt : Outport  Port=2
  wires:
  i_alpha/1 -> Subsystem/1(i_alpha)
  Subsystem/1(dia/dt) -> dia/dt/1
  i_beta/1 -> Subsystem1/1(i_beta)
  Subsystem1/1(dib/dt) -> dib/dt/1

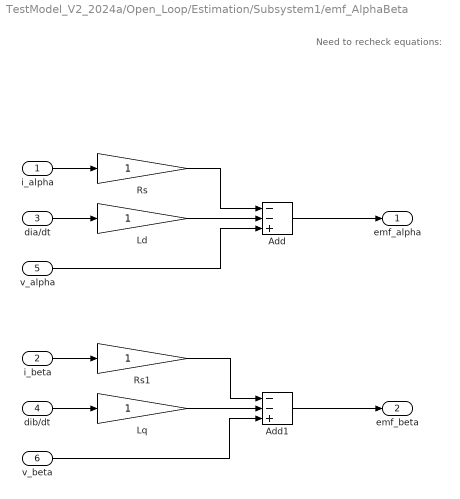
== system TestModel_V2_2024a/Open_Loop/Estimation/Subsystem1/emf_AlphaBeta ==
  note: Need to recheck equations:
  i_alpha : Inport
  i_beta : Inport  Port=2
  dia/dt : Inport  Port=3
  dib/dt : Inport  Port=4
  v_alpha : Inport  Port=5
  v_beta : Inport  Port=6
  Add : Sum  Inputs=--+
  Add1 : Sum  Inputs=--+
  Ld : Gain
  Lq : Gain
  Rs : Gain
  Rs1 : Gain
  emf_alpha : Outport
  emf_beta : Outport  Port=2
  wires:
  i_alpha/1 -> Rs/1
  dia/dt/1 -> Ld/1
  Ld/1 -> Add/2
  v_alpha/1 -> Add/3
  Rs/1 -> Add/1
  Add/1 -> emf_alpha/1
  Add1/1 -> emf_beta/1
  Rs1/1 -> Add1/1
  v_beta/1 -> Add1/3
  Lq/1 -> Add1/2
  dib/dt/1 -> Lq/1
  i_beta/1 -> Rs1/1

== system TestModel_V2_2024a/Open_Loop/Estimation/Subsystem1/di//dt/Subsystem ==
  i_alpha : Inport
  Add : Sum  Inputs=+-
  Gain : Gain  Gain=1/0.0001
  Unit Delay : UnitDelay  SampleTime=-1  HasFrameUpgradeWarning=on
  dia/dt : Outport
  wires:
  i_alpha/1 -> Unit Delay/1, Add/1
  Unit Delay/1 -> Add/2
  Add/1 -> Gain/1
  Gain/1 -> dia/dt/1

== system TestModel_V2_2024a/Open_Loop/Estimation/Subsystem1/di//dt/Subsystem1 ==
  i_beta : Inport
  Add : Sum  Inputs=+-
  Gain : Gain  Gain=1/0.0001
  Unit Delay : UnitDelay  SampleTime=-1  HasFrameUpgradeWarning=on
  dib/dt : Outport
  wires:
  Gain/1 -> dib/dt/1
  Add/1 -> Gain/1
  Unit Delay/1 -> Add/2
  i_beta/1 -> Add/1, Unit Delay/1

== matlab function TestModel_V2_2024a/Open_Loop/MATLAB Function1 ==
  data: speed_cmd input; y output; ramp_rate input; Ts input
%FileName: Ramp1
%Description: Function to ramp input u1 from output value u2. 
%Inputs: Any Signal Value
%Output: Ramp of input signal until the input value
%Created by: Devi Cheerla
%Created on: 21-08-2024
%Version no: 0.1

% function y = ramp1(u, data)
% u1=u;
% u2=data;
% dy=0.001*4;
% persistent yp;
% if isempty(yp)
%     yp=0;
% elseif (yp==yp && yp~=u2)
%     yp=u2;
% else
% end
% diff = u1-yp;
% 
% if diff>0
%     y=yp+dy;
% elseif diff<0
%     y=yp-dy;
% else
%     y=yp;
% end
% yp=y;
% 
% end


function y = speed_ramp(speed_cmd,ramp_rate,Ts)

persistent speed_ref

%Ts = 1e-6;
%Ts = 10e-3;

dN = ramp_rate * Ts;

if isempty(speed_ref)
    speed_ref = 0;
end

err = speed_cmd - speed_ref;

if abs(err) <= dN
    speed_ref = speed_cmd;
elseif err > 0
    speed_ref = speed_ref + dN;
else
    speed_ref = speed_ref - dN;
end

y = speed_ref;

end

== matlab function TestModel_V2_2024a/MATLAB Function ==
  data: V_Ph input; va output; vb output; vc output; t input
function [va,vb,vc] = fcn(V_Ph,t)

f = 50;
Vpk = sqrt(2)*V_Ph;


% for t=0:Ts:1/f
    va = Vpk*sin(2*pi*f*t);
    vb = Vpk*sin(2*pi*f*t - 2*pi/3);
    vc = Vpk*sin(2*pi*f*t + 2*pi/3);
% end
end

== matlab function TestModel_V2_2024a/Open_Loop/MATLAB Function2 ==
  data: speed_cmd input; y output; RampUpRate input; RampDownRate input; Ts input
%FileName: Ramp1
%Description: Function to ramp input u1 from output value u2. 
%Inputs: Any Signal Value
%Output: Ramp of input signal until the input value
%Created by: Devi Cheerla
%Created on: 21-08-2024
%Version no: 0.1

% function y = ramp1(u, data)
% u1=u;
% u2=data;
% dy=0.001*4;
% persistent yp;
% if isempty(yp)
%     yp=0;
% elseif (yp==yp && yp~=u2)
%     yp=u2;
% else
% end
% diff = u1-yp;
% 
% if diff>0
%     y=yp+dy;
% elseif diff<0
%     y=yp-dy;
% else
%     y=yp;
% end
% yp=y;
% 
% end


% function y = speed_ramp(speed_cmd,ramp_rate,Ts)
% 
% persistent speed_ref
% 
% % Ts = 1e-6;
% 
% dN = ramp_rate * Ts;
% 
% if isempty(speed_ref)
%     speed_ref = 0;
% end
% 
% err = speed_cmd - speed_ref;
% 
% if abs(err) <= dN
%     speed_ref = speed_cmd;
% elseif err > 0
%     speed_ref = speed_ref + dN;
% else
%     speed_ref = speed_ref - dN;
% end
% 
% y = speed_ref;
% 
% end

function y = speed_ramp(speed_cmd, RampUpRate, RampDownRate, Ts )

persistent speed_ref

% Ts = 1e-3;
% 
% RampUpRate   = 25;
% RampDownRate = 100;

if isempty(speed_ref)
    speed_ref = 0;
end

err = speed_cmd - speed_ref;

if err > 0

    dN = RampUpRate * Ts;

    if err <= dN
        speed_ref = speed_cmd;
    else
        speed_ref = speed_ref + dN;
    end

elseif err < 0

    dN = RampDownRate * Ts;

    if abs(err) <= dN
        speed_ref = speed_cmd;
    else
        speed_ref = speed_ref - dN;
    end

end

y = speed_ref;

end

== matlab function TestModel_V2_2024a/Open_Loop/Estimation/EBE_Observer ==
  data: i_alpha_hat output; i_beta_hat output; e_alpha_hat output; e_beta_hat output; v_alpha input; v_beta input; i_alpha_meas input; i_beta_meas input; Ts input; Rs input; L input; ki input; ke input
function [i_alpha_hat, i_beta_hat, e_alpha_hat, e_beta_hat] = ...
    ebe_step(v_alpha, v_beta, i_alpha_meas, i_beta_meas, Ts, Rs, L, ki, ke)

%#codegen
persistent i_alpha_hat_z i_beta_hat_z e_alpha_hat_z e_beta_hat_z
if isempty(i_alpha_hat_z)
    i_alpha_hat_z = i_alpha_meas;  % init at first sample
    i_beta_hat_z  = i_beta_meas;
    e_alpha_hat_z = 0.0;
    e_beta_hat_z  = 0.0;
end

% Errors
i_alpha_tilde = i_alpha_meas - i_alpha_hat_z;
i_beta_tilde  = i_beta_meas  - i_beta_hat_z;

% Current observer dynamics (discrete Euler)
di_alpha_hat = (1/L)*(v_alpha - Rs*i_alpha_hat_z - e_alpha_hat_z) + ki*i_alpha_tilde;
di_beta_hat  = (1/L)*(v_beta  - Rs*i_beta_hat_z  - e_beta_hat_z)  + ki*i_beta_tilde;

i_alpha_hat_next = i_alpha_hat_z + Ts*di_alpha_hat;
i_beta_hat_next  = i_beta_hat_z  + Ts*di_beta_hat;

% Back-EMF observer dynamics (discrete Euler)
de_alpha_hat = ke * i_alpha_tilde;
de_beta_hat  = ke * i_beta_tilde;

e_alpha_hat_next = e_alpha_hat_z + Ts*de_alpha_hat;
e_beta_hat_next  = e_beta_hat_z  + Ts*de_beta_hat;

% Optional: saturation on e_hat to avoid wind-up
E_MAX = 1e4; % set based on machine
e_alpha_hat_next = min(max(e_alpha_hat_next, -E_MAX), E_MAX);
e_beta_hat_next  = min(max(e_beta_hat_next,  -E_MAX),  E_MAX);

% Update state
i_alpha_hat_z = i_alpha_hat_next;
i_beta_hat_z  = i_beta_hat_next;
e_alpha_hat_z = e_alpha_hat_next;
e_beta_hat_z  = e_beta_hat_next;

% Outputs
i_alpha_hat = i_alpha_hat_z;
i_beta_hat  = i_beta_hat_z;
e_alpha_hat = e_alpha_hat_z;
e_beta_hat  = e_beta_hat_z;
end

== matlab function TestModel_V2_2024a/Open_Loop/MATLAB Function ==
  data: fe input; Vs output; Vs1 input; V_Boost input
function Vs = fcn(fe,Vs1,V_Boost)
%#codegen

% if fe<6
%     Vs=Vs1+V_Boost;
% else
%     Vs=Vs1;
% end

if fe<=0
    Vs = 0;
elseif fe>0 || fe<50
    Vs = V_Boost + (400-V_Boost)*fe/50;  %    V_Boost(1+(Vs1/V_Boost)-(fe/50))
else
    Vs= 400;
end

end

== matlab function TestModel_V2_2024a/Open_Loop/MATLAB Function5 ==
  data: u input; y output; data input
%FileName: Ramp1
%Description: Function to ramp input u1 from output value u2. 
%Inputs: Any Signal Value
%Output: Ramp of input signal until the input value
%Created by: Devi Cheerla
%Created on: 21-08-2024
%Version no: 0.1

function y = ramp1(u, data)
u1=u;
u2=data;
dy=0.001*4;
persistent yp;
if isempty(yp)
    yp=0;
elseif (yp==yp && yp~=u2)
    yp=u2;
else
end
diff = u1-yp;

if diff>0
    y=yp+dy;
elseif diff<0
    y=yp-dy;
else
    y=yp;
end
yp=y;

end

== matlab function TestModel_V2_2024a/Open_Loop/Estimation/MRAS_Observer ==
  data: v_alpha input; theta_est output; v_beta input; i_alpha input; i_beta input; Ts input; Rs input; Rr input; Ls input; Lr input; Lm input; Kp_SpdEst input; Ki_SpdEst input; omega_est output
function [theta_est, omega_est] = fcn(v_alpha, v_beta, i_alpha, i_beta, Ts, Rs, Rr, Ls, Lr, Lm, Kp_SpdEst, Ki_SpdEst)

Tr=Lr/Rr;    % Rotor time constant
sigma = 1 - (Lm^2)/(Ls*Lr);

%% Initialize States

% psi_ref = [0; 0];   % reference flux (alpha, beta)
% psi_est = [0; 0];   % estimated flux
% 
% omega_est = 0;
% theta_est = 0;
% 
% int_error = 0;

persistent psi_s_alpha psi_s_beta
persistent psi_r_est_alpha psi_r_est_beta
persistent omega_hat
persistent theta_hat
persistent int_error

if isempty(psi_s_alpha)
    psi_s_alpha = 0;
    psi_s_beta = 0;
    psi_r_est_alpha = 0;
    psi_r_est_beta = 0;
    omega_hat = 0;
    theta_hat = 0;
    int_error = 0;
end

%% Reference Model

% Inputs: Valpha, Vbeta, Ialpha, Ibeta

% psi_ref_dot = [v_alpha; v_beta] - Rs * [i_alpha; i_beta];
% psi_ref = psi_ref + psi_ref_dot * Ts;

psi_s_alpha_dot = v_alpha - Rs * i_alpha;
psi_s_beta_dot =  v_beta  - Rs * i_beta;
psi_s_alpha = psi_s_alpha + psi_s_alpha_dot * Ts;
psi_s_beta  = psi_s_beta + psi_s_beta_dot * Ts;

%% Rotor Flux Reference

psi_r_ref_alpha = (Lr/Lm) * (psi_s_alpha - sigma*Ls*i_alpha);

psi_r_ref_beta = (Lr/Lm) * (psi_s_beta - sigma*Ls*i_beta);

%% Adaptive Model 

% psi_est_dot = (Lm/Tr) * [i_alpha; i_beta] ...
%               - (1/Tr) * psi_est ...
%               - omega_est * [0 -1; 1 0] * psi_est;
% 
% psi_est = psi_est + psi_est_dot * Ts;

psi_r_est_alpha_dot = (Lm/Tr)*i_alpha - (1/Tr)*psi_r_est_alpha + omega_hat*psi_r_est_beta;

psi_r_est_beta_dot = (Lm/Tr)*i_beta - (1/Tr)*psi_r_est_beta - omega_hat*psi_r_est_alpha;

psi_r_est_alpha = psi_r_est_alpha + psi_r_est_alpha_dot*Ts;

psi_r_est_beta = psi_r_est_beta + psi_r_est_beta_dot*Ts;

%% Error Calculation

% e = psi_ref(1) * psi_est(2) - psi_ref(2) * psi_est(1);    % Error Calculation

e = psi_r_ref_alpha*psi_r_est_beta - psi_r_ref_beta *psi_r_est_alpha;

%% Speed Estimation

int_error = int_error + e * Ts;

% Anti-windup
INT_LIMIT = 500;

if int_error > INT_LIMIT
    int_error = INT_LIMIT;
elseif int_error < -INT_LIMIT
    int_error = -INT_LIMIT;
end

omega_hat = Kp_SpdEst * e + Ki_SpdEst * int_error;

%Speed Limit

OMEGA_MAX = 1000;

if omega_hat > OMEGA_MAX
    omega_hat = OMEGA_MAX;
elseif omega_hat < -OMEGA_MAX
    omega_hat = -OMEGA_MAX;
end


%% Angle Update

% theta_est = theta_est + omega_est * Ts;

theta_hat = theta_hat + omega_hat*Ts;
%% Wrap Angle

%theta_est_obs = mod(theta_est, 2*pi);

theta_hat = mod(theta_hat,2*pi);

%% Outputs

theta_est = theta_hat;

omega_est = omega_hat;

end
